simulink model "pendule_inv_echant_etu"  (R2022a)
settings: Solver=VariableStepAuto  StartTime=0.0  StopTime=10.0  RelTol=1e-3
values from neighbouring files (symbols this model uses):
  delta_t = 0.4    [simu_pendule_inv_echant_etu.m]
  g = 9.81    [simu_pendule_inv_capteur_etu.m]    (also in simu_pendule_inv_echant_etu.m; simu_pendule_inv_etu.m)
  K = [10 1]    [simu_pendule_inv_capteur_etu.m]    (also in simu_pendule_inv_echant_etu.m = [30 10]; simu_pendule_inv_etu.m = [30 10])
  l = 10    [simu_pendule_inv_capteur_etu.m]    (also in simu_pendule_inv_echant_etu.m; simu_pendule_inv_etu.m)
  ue = 0    [simu_pendule_inv_capteur_etu.m]    (also in simu_pendule_inv_echant_etu.m; simu_pendule_inv_etu.m)
  x0 = [pi/20 0]'    [simu_pendule_inv_capteur_etu.m]    (also in simu_pendule_inv_echant_etu.m; simu_pendule_inv_etu.m = [pi/10 0]')
  xe = [0 0]'    [simu_pendule_inv_capteur_etu.m]    (also in simu_pendule_inv_echant_etu.m; simu_pendule_inv_etu.m)
undefined symbols (not defined in the file or in its folder): DiscIntNeverNeededParam
settings Model: Creator=paul  LastModifiedBy=paul
settings ModelReferenceCC: EnableRefExpFcnMdlSchedulingChecks=off
settings RTWCC: Description=Generic Real-Time Target

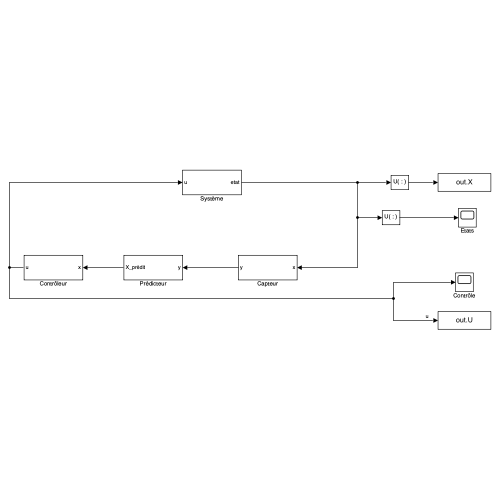
[thumbnail: Simulink's stored preview of the top-level diagram]
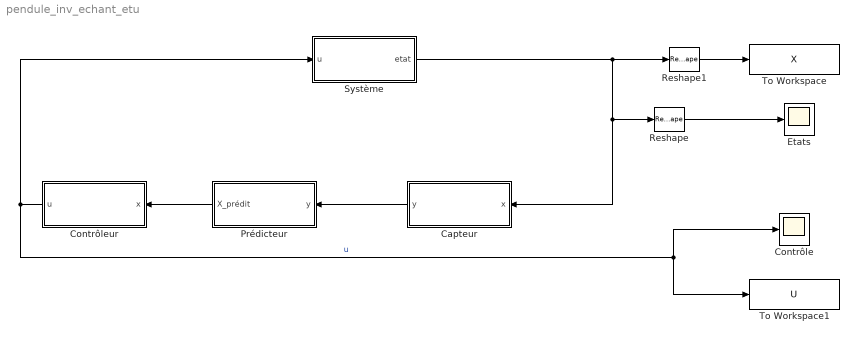
== system pendule_inv_echant_etu ==
  Capteur : Subsystem
  Contrôle : Scope
  Contrôleur : Subsystem
  Etats : Scope
  Prédicteur : Subsystem
  Reshape : Reshape
  Reshape1 : Reshape
  Système : Subsystem
  To Workspace : ToWorkspace  VariableName=X  SaveFormat=Timeseries  SampleTime=-1
  To Workspace1 : ToWorkspace  VariableName=U  SaveFormat=Timeseries  SampleTime=-1
  wires:
  Reshape/1 -> Etats/1
  Reshape1/1 -> To Workspace/1
  Système/1(etat) -> Capteur/1(x), Reshape/1, Reshape1/1
  Contrôleur/1(u) -> Système/1(u), To Workspace1/1, Contrôle/1  "u"
  Prédicteur/1(X_prédit) -> Contrôleur/1(x)
  Capteur/1(y) -> Prédicteur/1(y)

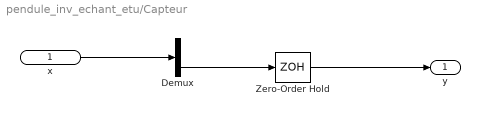
== system pendule_inv_echant_etu/Capteur ==
  x : Inport
  Demux : Demux  Outputs=2
  Zero-Order Hold : ZeroOrderHold  SampleTime=delta_t
  y : Outport
  wires:
  x/1 -> Demux/1
  Demux/2 -> Zero-Order Hold/1
  Zero-Order Hold/1 -> y/1

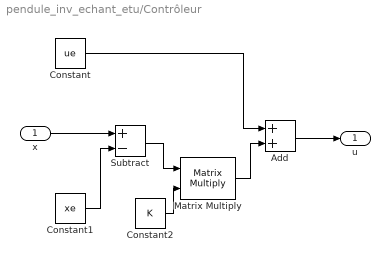
== system pendule_inv_echant_etu/Contrôleur ==
  x : Inport
  Add : Sum
  Constant : Constant  Value=ue
  Constant1 : Constant  Value=xe
  Constant2 : Constant  Value=K
  Matrix Multiply : Product  Multiplication=Matrix(*)
  Subtract : Sum  Inputs=+-
  u : Outport
  wires:
  x/1 -> Subtract/1
  Constant1/1 -> Subtract/2
  Subtract/1 -> Matrix Multiply/1
  Constant/1 -> Add/1
  Matrix Multiply/1 -> Add/2
  Add/1 -> u/1
  Constant2/1 -> Matrix Multiply/2

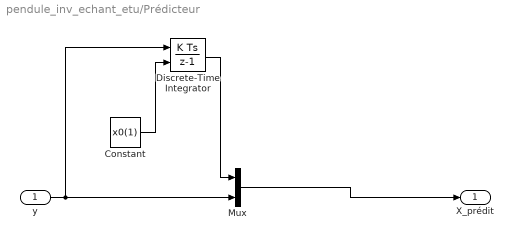
== system pendule_inv_echant_etu/Prédicteur ==
  y : Inport
  Constant : Constant  Value=x0(1)
  Discrete-Time Integrator : DiscreteIntegrator  InitialConditionSource=external  SampleTime=-1  ICPrevOutput=DiscIntNeverNeededParam  ICPrevScaledInput=DiscIntNeverNeededParam
  Mux : Mux  Inputs=2
  X_prédit : Outport
  wires:
  y/1 -> Discrete-Time Integrator/1, Mux/2
  Mux/1 -> X_prédit/1
  Discrete-Time Integrator/1 -> Mux/1
  Constant/1 -> Discrete-Time Integrator/2

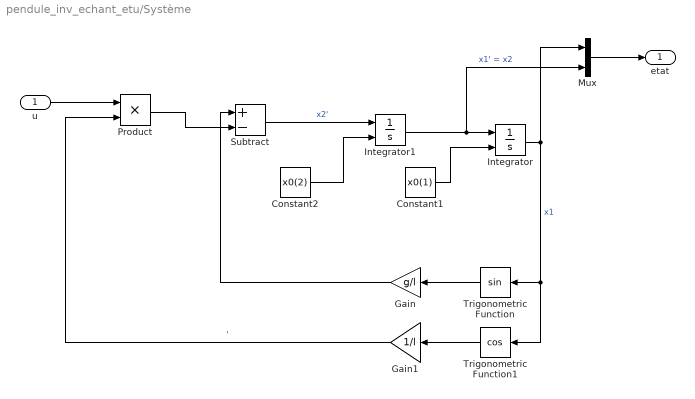
== system pendule_inv_echant_etu/Système ==
  u : Inport
  Constant1 : Constant  Value=x0(1)
  Constant2 : Constant  Value=x0(2)
  Gain : Gain  Gain=g/l
  Gain1 : Gain  Gain=1/l
  Integrator : Integrator  InitialConditionSource=external
  Integrator1 : Integrator  InitialConditionSource=external
  Mux : Mux  Inputs=2
  Product : Product
  Subtract : Sum  Inputs=+-
  Trigonometric Function : Trigonometry
  Trigonometric Function1 : Trigonometry  Operator=cos
  etat : Outport
  wires:
  Integrator/1 -> Mux/1, Trigonometric Function/1, Trigonometric Function1/1  "x1"
  Integrator1/1 -> Mux/2, Integrator/1  "x1' = x2"
  Trigonometric Function/1 -> Gain/1
  Trigonometric Function1/1 -> Gain1/1
  u/1 -> Product/1
  Subtract/1 -> Integrator1/1  "x2'"
  Gain1/1 -> Product/2  "'"
  Constant1/1 -> Integrator/2
  Constant2/1 -> Integrator1/2
  Mux/1 -> etat/1
  Gain/1 -> Subtract/1
  Product/1 -> Subtract/2
